simulink model "hw8_two_tanks"  (R2014a)
settings: Solver=ode45  StartTime=0.0  StopTime=4  RelTol=1e-3
settings Model: Creator=feisele  LastModifiedBy=feisele

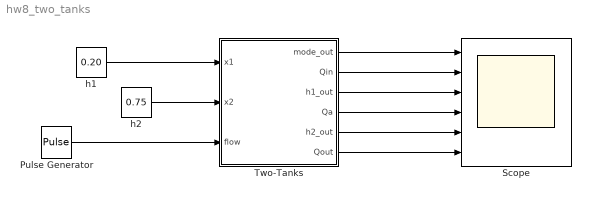
== system hw8_two_tanks ==
  Pulse Generator : DiscretePulseGenerator  PulseType=Time based  Period=1  PulseWidth=50
  Scope : Scope  NumInputPorts=6
      settings: ShowLegends=on  TimeRange=4  YMin=-2~-0.01~0~-0.1~-0.5~-0.05  YMax=3~0.1~1~0.1~0.5~0.15
  Two-Tanks : Stateflow chart  TreatAsAtomicUnit=on
  h1 : Constant  Value=0.20
  h2 : Constant  Value=0.75
  wires:
  h1/1 -> Two-Tanks/1(x1)
  h2/1 -> Two-Tanks/2(x2)
  Pulse Generator/1 -> Two-Tanks/3(flow)
  Two-Tanks/1(mode_out) -> Scope/1
  Two-Tanks/2(Qin) -> Scope/2
  Two-Tanks/3(h1_out) -> Scope/3
  Two-Tanks/4(Qa) -> Scope/4
  Two-Tanks/5(h2_out) -> Scope/5
  Two-Tanks/6(Qout) -> Scope/6

== stateflow chart hw8_two_tanks/Two-Tanks ==
  settings: updateMethod=CONTINUOUS
  state From_tank_1
    during:
    % derivatives
    h1_dot = (qi() - qa_from_tank(h1, h)) / A;
    h2_dot = (qa_from_tank(h1, h) - qo()) / A;
    % output
    mode_out = 1;
    Qin = qi();
    Qa = qa_from_tank(h1, h);
    Qout = qo() ;
    h1_out = h1;
    h2_out = h2;
  state Separated
    during:
    % derivatives
    h1_dot = qi() / A;
    h2_dot = - qo() / A;
    %output
    mode_out = 0;
    Qin =  qi();
    Qout = qo() ;
    h1_out = h1;
    h2_out = h2;
  state Balancing
    during:
    % derivatives
    h1_dot = (qi() - qa_balancing(h1, h2)) / A;
    h2_dot = (qa_balancing(h1, h2) - qo()) / A;
    % output
    mode_out = 2;
    Qin = qi();
    Qa = qa_balancing(h1, h2);
    Qout = qo() ;
    h1_out = h1;
    h2_out = h2;
  state From_tank_2
    during:
    % derivatives
    h1_dot = (qi() - qa_from_tank(h2, h)) / A;
    h2_dot = (qa_from_tank(h2, h) - qo()) / A;
    % output
    mode_out = -1;
    Qin = qi();
    Qa = qa_from_tank(h2, h);
    Qout = qo() ;
    h1_out = h1;
    h2_out = h2;
  (default) -> Separated : { h1 = x1 , h2 = x2}
  Separated -> (junction 18) [order 1]
  From_tank_1 -> (junction 17) [order 1]
  From_tank_1 -> (junction 19) [order 2]
  Separated -> (junction 20) [order 2]
  Separated -> (junction 19) [order 3]
  (junction 17) -> Separated : [h1 < h && h2 < h]
  (junction 18) -> From_tank_1 : [h1 > h && h2 < h]
  From_tank_1 -> (junction 20) [order 3]
  From_tank_2 -> (junction 17) [order 1]
  Balancing -> (junction 18) [order 2]
  Balancing -> (junction 17) [order 1]
  From_tank_2 -> (junction 18) [order 2]
  (junction 20) -> Balancing : [h1 > h && h2 > h]
  Balancing -> (junction 19) [order 3]
  (junction 19) -> From_tank_2 : [h1 < h && h2 > h]
  From_tank_2 -> (junction 20) [order 3]
  data: q function_output; q function_output; ha function_input; hb function_input; qa function_output; ha function_input; hb function_input; q function_output; mode_out output; h1 local double; h constant double =0.3; h2 local double; Qin output double; h1_out output; Qa output double; h2_out output; A constant double =0.0154; Qout output double; x1 input double; x2 input double; rho constant double =1000; g constant double =9.81; Kin constant double =0.06; Ka constant double =0.001; Kout constant double =0.001; flow input double
  data h1 settings: updateMethod=SF_CONTINUOUS_TIME_DATA
  data h settings: updateMethod=SF_CONTINUOUS_TIME_DATA
  data h2 settings: updateMethod=SF_CONTINUOUS_TIME_DATA
  function q=qi:
    | function q=qi()
    | %%QO Compute output flow rate from tank 2
    | % A negative flow value should be avoided.
    | % It would be non-physical.
    | q = Kin * flow;
  function q=qo:
    | function q=qo()
    | %%QO Compute output flow rate from tank 2
    | % A negative flow rate is allowed so the 
    | % solver can detect zero-crossing.
    | q = sign(h2) * Kout * sqrt(rho * g * abs(h2));
  function qa=qa_from_tank(ha, hb):
    | function qa=qa_from_tank(ha, hb)
    | %%Q_A_FROM_TANK Compute flow rate from higher tank 
    | % A negative flow rate is allowed for the
    | % solver to detect zero crossing.
    | delta = ha - hb;
    | qa = sign(delta) * Ka * sqrt(rho * g * abs(delta));
  function q=qa_balancing(ha, hb):
    | function q=qa_balancing(ha, hb)
    | %%QA_BALANCING Compute balanced flow between tanks 1 and 2
    | % A negative flow rate indicates flow from 2 to 1.
    | delta = ha - hb;
    | q = sign(delta) * Ka * sqrt(rho * g * abs(delta));
